simulink model "scheme2"  (R2014a)
settings: Solver=ode45  StartTime=0.0  StopTime=0.4  RelTol=1e-3
settings Model: Creator=User  LastModifiedBy=Анастасия

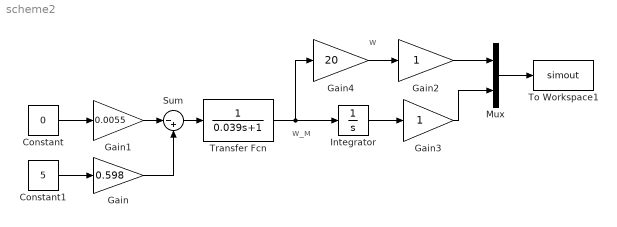
== system scheme2 ==
  note: w
  note: w_м
  Constant : Constant  Value=0
  Constant1 : Constant  Value=5
  Gain : Gain  Gain=0.598
  Gain1 : Gain  Gain=0.0055
  Gain2 : Gain
  Gain3 : Gain
  Gain4 : Gain  Gain=20
  Integrator : Integrator
  Mux : Mux  Inputs=2
  Sum : Sum  Inputs=|-+
  To Workspace1 : ToWorkspace  VariableName=simout  SaveFormat=Timeseries  SampleTime=-1
  Transfer Fcn : TransferFcn  Denominator=[0.039 1]
  wires:
  Sum/1 -> Transfer Fcn/1
  Integrator/1 -> Gain3/1
  Constant1/1 -> Gain/1
  Constant/1 -> Gain1/1
  Gain/1 -> Sum/2
  Gain1/1 -> Sum/1
  Transfer Fcn/1 -> Integrator/1, Gain4/1
  Gain2/1 -> Mux/1
  Gain3/1 -> Mux/2
  Mux/1 -> To Workspace1/1
  Gain4/1 -> Gain2/1
